simulink model "queseyo"  (R2015a)
settings: Solver=ode4  StartTime=0.0  StopTime=10.0  FixedStep=0.001  RelTol=1e-3
values from neighbouring files (symbols this model uses):
  A = [[   0      1         0         0         0         0] ... (first row only)    [test2.m]    (also in test3.m = [[   0      0         0         1         0         0]; test4.m = [[   0      0         0         1         0         0]; test5.m = [[zeros(2,2) eye(2)];[dg zeros(2,2)]])
  B = [0 22.07202 0 -151.371141 0 -56.32414]'    [test2.m]    (also in test3.m = [0 0 0 -0.6070 1.4984 -0.2839]'; test4.m = [0 0 0 -0.6070 1.4984 -0.2839]'; test5.m = [[zeros(2,1)]; [di*h]])
  g = 9.8    [test2.m]    (also in test3.m; test4.m; test5.m = [[-f1 0];[0 -f2]])
  K = aux2*Wr_canonica*inv(Wr)    [test2.m]    (also in test3.m; test4.m = acker(A, B, pk); test5.m = acker(A, B, pk))
  L = inv(Wo)*Wo_canonica*aux2'    [test2.m]    (also in test3.m; test4.m = acker(A', -C', pl)'; test5.m = acker(A', -C', pl)')
  n0 = M0+M1+M2    (= 0.079)    [test2.m]
  n1 = M1*L1+M2*L2    (= 0.00186)    [test2.m]
  n3 = M2*L2    (= 0.00024)    [test2.m]
  n4 = M2*L1*L2    (= 2.16e-05)    [test2.m]
  n5 = M2*L2^2    (= 3.6e-06)    [test2.m]
  n6 = M1*L1^2+M2*L1^2    (= 0.0002754)    [test2.m]
  r = 0    [test2.m]    (also in test3.m; test4.m; test5.m)
settings Model: Creator=Gonza  LastModifiedBy=joseg
settings SolverCC: AlgebraicLoopSolver=LineSearch

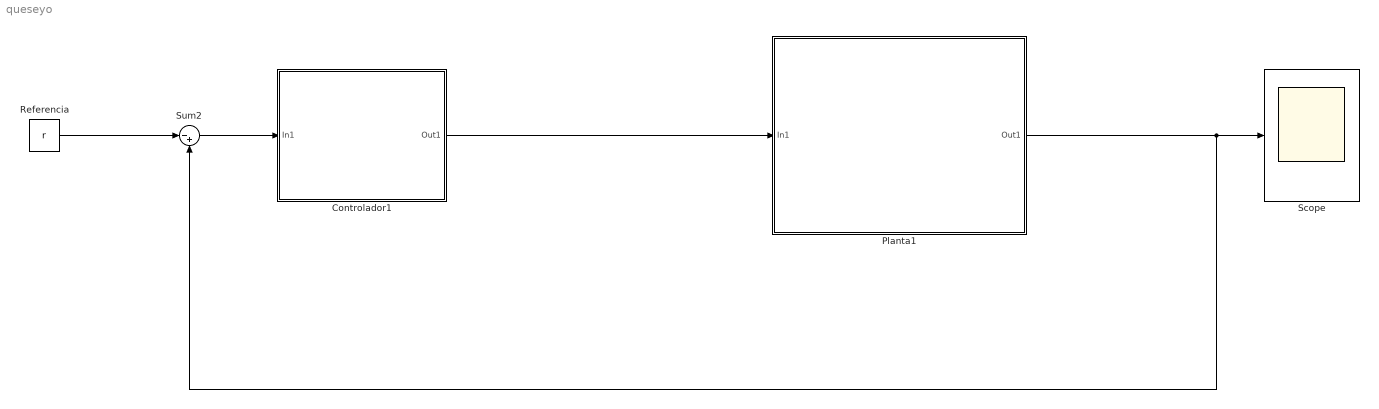
== system queseyo ==
  Controlador1 : Subsystem
  Planta1 : Subsystem
  Referencia : Constant  Value=r
  Scope : Scope
      settings: TimeRange=10  YMin=-1  YMax=1.5
  Sum2 : Sum  Inputs=|-+
  wires:
  Planta1/1(Out1) -> Sum2/2, Scope/1
  Referencia/1 -> Sum2/1
  Sum2/1 -> Controlador1/1(In1)
  Controlador1/1(Out1) -> Planta1/1(In1)

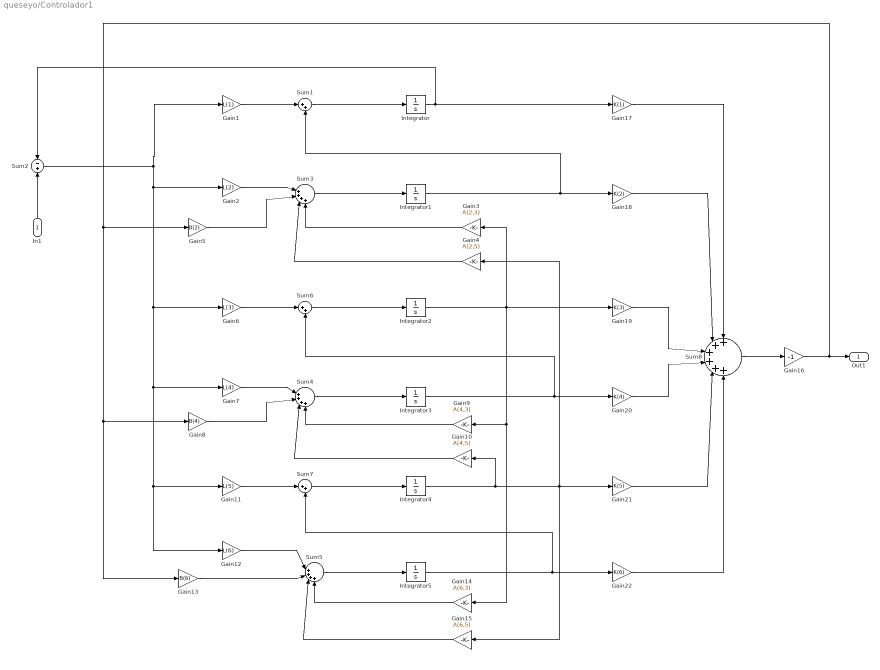
== system queseyo/Controlador1 ==
  In1 : Inport
  Gain1 : Gain  Gain=L(1)
  Gain10 : Gain  Gain=A(4,5)
  Gain11 : Gain  Gain=L(5)
  Gain12 : Gain  Gain=L(6)
  Gain13 : Gain  Gain=B(6)
  Gain14 : Gain  Gain=A(6,3)
  Gain15 : Gain  Gain=A(6,5)
  Gain16 : Gain  Gain=-1
  Gain17 : Gain  Gain=K(1)
  Gain18 : Gain  Gain=K(2)
  Gain19 : Gain  Gain=K(3)
  Gain2 : Gain  Gain=L(2)
  Gain20 : Gain  Gain=K(4)
  Gain21 : Gain  Gain=K(5)
  Gain22 : Gain  Gain=K(6)
  Gain3 : Gain  Gain=A(2,3)
  Gain4 : Gain  Gain=A(2,5)
  Gain5 : Gain  Gain=B(2)
  Gain6 : Gain  Gain=L(3)
  Gain7 : Gain  Gain=L(4)
  Gain8 : Gain  Gain=B(4)
  Gain9 : Gain  Gain=A(4,3)
  Integrator{,1..5} (6 alike) : Integrator
  Sum1 : Sum  Inputs=|++
  Sum2 : Sum  Inputs=-+
  Sum3 : Sum  Inputs=||++++
  Sum4 : Sum  Inputs=||++++
  Sum5 : Sum  Inputs=||++++
  Sum6 : Sum  Inputs=|++
  Sum7 : Sum  Inputs=|++
  Sum8 : Sum  Inputs=+|+|+|+|+|+
  Out1 : Outport
  wires:
  Sum1/1 -> Integrator/1
  Integrator1/1 -> Gain18/1, Sum1/2
  Gain1/1 -> Sum1/1
  Sum2/1 -> Gain1/1, Gain12/1, Gain11/1, Gain7/1, Gain6/1, Gain2/1
  Sum3/1 -> Integrator1/1
  Gain2/1 -> Sum3/1
  Integrator4/1 -> Gain21/1, Gain4/1, Gain15/1, Gain10/1
  Integrator2/1 -> Gain19/1, Gain14/1, Gain9/1, Gain3/1
  Gain4/1 -> Sum3/3
  Gain3/1 -> Sum3/4
  Gain5/1 -> Sum3/2
  Sum6/1 -> Integrator2/1
  Integrator3/1 -> Gain20/1, Sum6/2
  Gain6/1 -> Sum6/1
  Sum4/1 -> Integrator3/1
  Gain7/1 -> Sum4/1
  Gain8/1 -> Sum4/2
  Gain9/1 -> Sum4/4
  Gain10/1 -> Sum4/3
  Sum7/1 -> Integrator4/1
  Integrator5/1 -> Gain22/1, Sum7/2
  Gain11/1 -> Sum7/1
  Sum5/1 -> Integrator5/1
  Gain12/1 -> Sum5/1
  Gain13/1 -> Sum5/2
  Gain14/1 -> Sum5/4
  Gain15/1 -> Sum5/3
  In1/1 -> Sum2/2
  Integrator/1 -> Gain17/1, Sum2/1
  Gain16/1 -> Gain13/1, Gain8/1, Gain5/1, Out1/1
  Sum8/1 -> Gain16/1
  Gain17/1 -> Sum8/1
  Gain18/1 -> Sum8/2
  Gain19/1 -> Sum8/3
  Gain20/1 -> Sum8/4
  Gain21/1 -> Sum8/5
  Gain22/1 -> Sum8/6

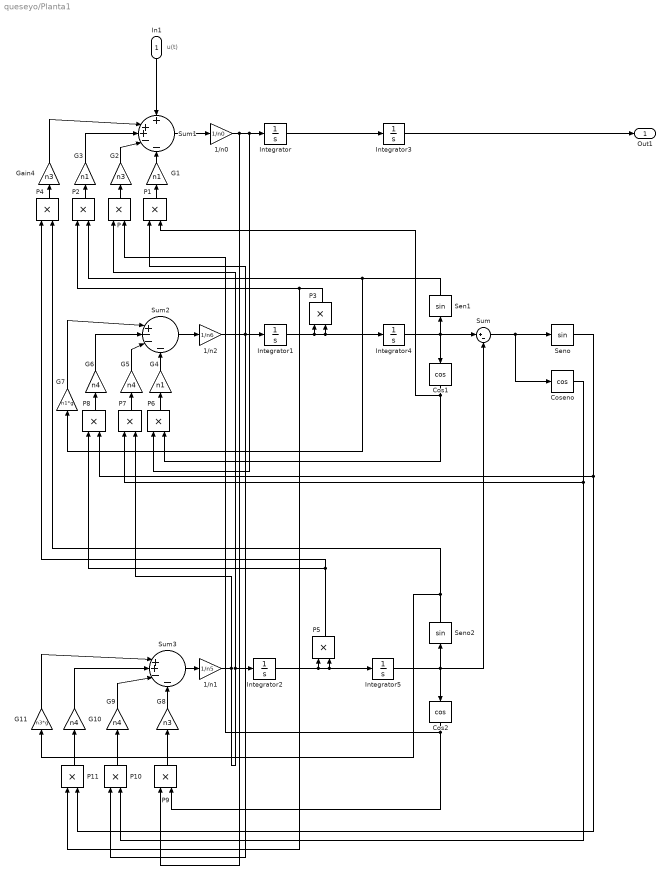
== system queseyo/Planta1 ==
  note: u(t)
  In1 : Inport
  1/n0 : Gain  Gain=1/n0
  1/n1 : Gain  Gain=1/n5
  1/n2 : Gain  Gain=1/n6
  Cos1 : Trigonometry  Operator=cos
  Cos2 : Trigonometry  Operator=cos
  Coseno : Trigonometry  Operator=cos
  G1 : Gain  Gain=n1
  G{5..6,9..10} (4 alike) : Gain  Gain=n4
  G11 : Gain  Gain=n3*g
  G2 : Gain  Gain=n3
  G3 : Gain  Gain=n1
  G4 : Gain  Gain=n1
  G7 : Gain  Gain=n1*g
  G8 : Gain  Gain=n3
  Gain4 : Gain  Gain=n3
  Integrator{,1..5} (6 alike) : Integrator
  P{,1..11} (12 alike) : Product
  Sen1 : Trigonometry
  Seno : Trigonometry
  Seno2 : Trigonometry
  Sum : Sum  Inputs=|+-
  Sum1 : Sum  Inputs=+|++-|-
  Sum2 : Sum  Inputs=||+--|-
  Sum3 : Sum  Inputs=||++-|-
  Out1 : Outport
  wires:
  Integrator/1 -> Integrator3/1
  Integrator1/1 -> P3/1, P3/2, Integrator4/1
  Integrator2/1 -> P5/1, P5/2, Integrator5/1
  Integrator4/1 -> Cos1/1, Sen1/1, Sum/1
  Integrator5/1 -> Cos2/1, Seno2/1, Sum/2
  Sum/1 -> Coseno/1, Seno/1
  Integrator3/1 -> Out1/1
  In1/1 -> Sum1/1
  Sum1/1 -> 1/n0/1
  1/n0/1 -> P9/1, P6/1, Integrator/1
  G1/1 -> Sum1/5
  P1/1 -> G1/1
  Cos1/1 -> P1/2, P6/2
  Sum2/1 -> 1/n2/1
  P/1 -> G2/1
  Cos2/1 -> P9/2, P/2
  G2/1 -> Sum1/4
  Sum3/1 -> 1/n1/1
  G3/1 -> Sum1/3
  P2/1 -> G3/1
  Sen1/1 -> P2/2, G7/1
  P3/1 -> P2/1, P11/1
  P4/1 -> Gain4/1
  Gain4/1 -> Sum1/2
  Seno2/1 -> G11/1, P4/2
  P5/1 -> P8/1, P4/1
  1/n2/1 -> P10/1, Integrator1/1, P1/1
  G4/1 -> Sum2/4
  P6/1 -> G4/1
  G5/1 -> Sum2/3
  P7/1 -> G5/1
  Coseno/1 -> P10/2, P7/1
  P8/1 -> G6/1
  Seno/1 -> P8/2, P11/2
  G6/1 -> Sum2/2
  G7/1 -> Sum2/1
  1/n1/1 -> Integrator2/1, P/1, P7/2
  G8/1 -> Sum3/4
  P9/1 -> G8/1
  G9/1 -> Sum3/3
  P10/1 -> G9/1
  G10/1 -> Sum3/2
  P11/1 -> G10/1
  G11/1 -> Sum3/1
